simulink library "INT_ACSwt_VD"  (R2016b)
settings: Solver=VariableStepAuto  StartTime=0.0  StopTime=10.0  RelTol=1e-3
settings Model: Creator=胡炎林  LastModifiedBy=胡炎林

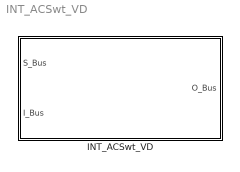
== system INT_ACSwt_VD ==
  INT_ACSwt_VD : Subsystem

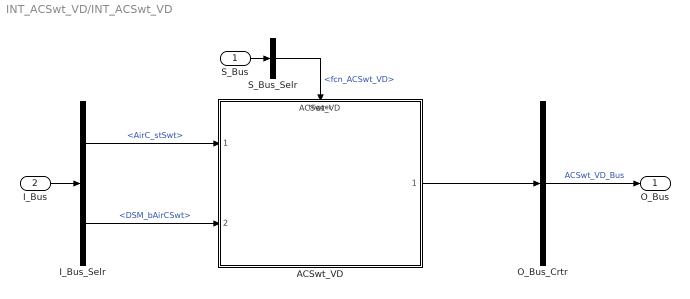
== system INT_ACSwt_VD/INT_ACSwt_VD ==
  S_Bus : Inport
  I_Bus : Inport  Port=2
  ACSwt_VD : ModelReference  ModelNameDialog=ACSwt_VD  SimulationMode=Normal  ModelReferenceVersion=1.10  TriggerPortName=function  TriggerPortTriggerType=function-call  TriggerPortStatesWhenEnabling=held
  I_Bus_Selr : BusSelector  OutputSignals=AirC_stSwt,DSM_bAirCSwt
  O_Bus_Crtr : BusCreator  Inputs=1
  S_Bus_Selr : BusSelector  OutputSignals=fcn_ACSwt_VD
  O_Bus : Outport
  wires:
  S_Bus_Selr/1 -> ACSwt_VD/Trigger  "<fcn_ACSwt_VD>"
  S_Bus/1 -> S_Bus_Selr/1
  I_Bus/1 -> I_Bus_Selr/1
  I_Bus_Selr/1 -> ACSwt_VD/1  "<AirC_stSwt>"
  I_Bus_Selr/2 -> ACSwt_VD/2  "<DSM_bAirCSwt>"
  O_Bus_Crtr/1 -> O_Bus/1  "ACSwt_VD_Bus"
  ACSwt_VD/1 -> O_Bus_Crtr/1
